simulink model "Debug_STEVAL_BMS _114"  (R2025b)
settings: Solver=FixedStepAuto  StartTime=0.0  StopTime=inf  MaxStep=.01  RelTol=1e-3  EnableMultiTasking=on
PreLoadFcn:
  | %setup_sil;
  | setup_pil;
InitFcn:
  | battery_init;
  | Full_Charge_Volt=4.2; % unit volts
  | Cutoff_Volt=3; % unit volts
  | Delta=.02;
  | ContactorTime=20;
  | ContactorTimeOut=100;
  | High_TempLim=333;
  | Low_TempLim=263;
  | Sensor_Fault_Treshold=.02;
  | CurrentTimeout=1;
  | Allowed_Delta=.04;
  | Bal_On_Time=30;
  | Bal_Off_Time=5;
  | BalNotAct_Time=10;
libraries: simulink x7, stm32blockslib x1, stm32f4xxblockslib x1
settings Model: DataDictionary=Needed_Buses.sldd  STM32="{\"DigitalPortWrite\":[{\"ID\":\"MCU_CODE:12\"},{\"ID\":\"MCU_CODE_Copy:132\"},{\"ID\":\"BMS_PIL_Wrapper:132\"},{\"ID\":\"BMS_MCU_CODE:1376\"}],\"DigitalPortRead\":[{\"ID\":\"MCU_CODE_Copy:131\"},{\"ID\":\"BMS_PIL_Wrapper:131\"}],\"SPIControllerTransfer\":{\"ID\":\"BMS_MCU_CODE:732\"}}"  SILPILSystemUnderTest=refmodels  CodeVerificationMode=processor-in-the-loop (pil)  Creator=Odonata-KJ  LastModifiedBy=Odonata-KJ
settings SolverCC: AutoInsertRateTranBlk=on
settings DataIOCC: SaveOutput=off  SaveTime=off
settings OptimizationCC: EnhancedBackFolding=on  PassReuseOutputArgsAs=Individual arguments  ZeroExternalMemoryAtStartup=off  ZeroInternalMemoryAtStartup=off  MaxStackSize=512  OptimizeBlockOrder=speed  DifferentSizesBufferReuse=on  OptimizationCustomize=off  EfficientTunableParamExpr=on
settings DebuggingCC: ParameterTunabilityLossMsg=error  SFUnexpectedBacktrackingDiag=warning  SFNoUnconditionalDefaultTransitionDiag=warning  UnderSpecifiedDimensionMsg=warning
settings HardwareCC: ProdBitPerPointer=32.0  ProdBitPerSizeT=32.0  ProdBitPerPtrDiffT=32.0  ProdLargestAtomicInteger=Long  ProdLargestAtomicFloat=Double  ProdWordSize=32.0  ProdLongLongMode=on  ProdHWDeviceType=ARM Compatible->ARM Cortex-M  TargetLargestAtomicInteger=Long  TargetLargestAtomicFloat=Double  TargetIntDivRoundTo=Zero  TargetEndianess=LittleEndian  TargetHWDeviceType=ARM Compatible->ARM Cortex-M
settings SFSimCC: MATLABDynamicMemAlloc=off
settings RTWCC: SystemTargetFile=ert.tlc  HardwareBoard=STM32F4xx Based  TemplateMakefile=ert_default_tmf  GenerateReport=on  Toolchain=GNU Tools for ARM Embedded Processors  BuildConfiguration=Debug  LaunchReport=on  PortableWordSizes=on  Description=Embedded Coder
settings CodeAppCC: ForceParamTrailComments=on  IgnoreCustomStorageClasses=off  OperatorAnnotations=on  SimulinkDataObjDesc=on  SFDataObjDesc=on  InsertBlockDesc=on  EnableCustomComments=on
settings ERTTargetCC: ExtModeTransport=3.0  ExtModeStaticAlloc=on  ExtModeStaticAllocSize=2048.0  ExtModeMexFile=ext_xcp  ExtModeIntrfLevel=Level2 - Open  InlinedParameterPlacement=Hierarchical  TargetLangStandard=C99 (ISO)

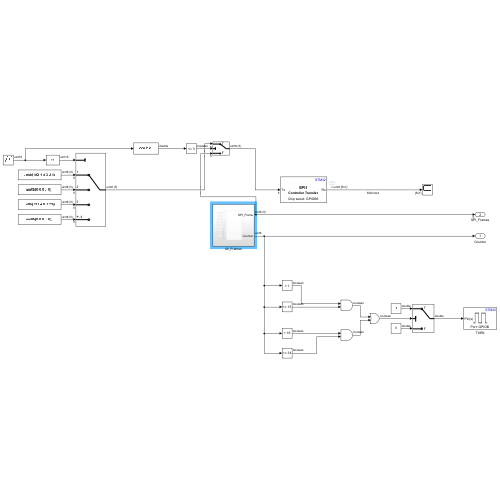
[thumbnail: Simulink's stored preview of the top-level diagram]
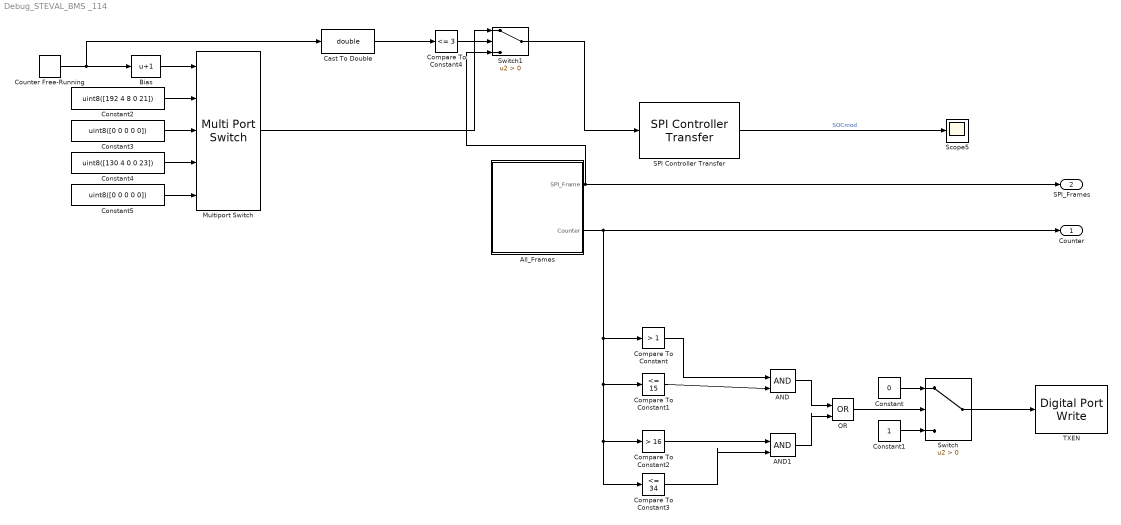
== system Debug_STEVAL_BMS _114 ==
  AND : Logic  IconShape=distinctive  AllPortsSameDT=off  OutDataTypeStr=boolean
  AND1 : Logic  IconShape=distinctive  AllPortsSameDT=off  OutDataTypeStr=boolean
  All_Frames : Subsystem
  Bias : Bias  Bias=1  SaturateOnIntegerOverflow=off
  Cast To Double : DataTypeConversion  OutDataTypeStr=double  SaturateOnIntegerOverflow=off  RndMeth=Floor
  Compare To Constant : simulink/Logic and Bit Operations/Compare To Constant  relop=>  const=1  OutDataTypeStr=boolean
  Compare To Constant1 : simulink/Logic and Bit Operations/Compare To Constant  relop=<=  const=15  OutDataTypeStr=boolean
  Compare To Constant2 : simulink/Logic and Bit Operations/Compare To Constant  relop=>  const=16  OutDataTypeStr=boolean
  Compare To Constant3 : simulink/Logic and Bit Operations/Compare To Constant  relop=<=  const=34  OutDataTypeStr=boolean
  Compare To Constant4 : simulink/Logic and Bit Operations/Compare To Constant  relop=<=  const=3  OutDataTypeStr=boolean
  Constant : Constant  Value=0
  Constant1 : Constant
  Constant2 : Constant  Value=uint8([192 4 8 0 21])
  Constant3 : Constant  Value=uint8([0 0 0 0 0])
  Constant4 : Constant  Value=uint8([130 4 0 0 23])
  Constant5 : Constant  Value=uint8([0 0 0 0 0])
  Counter Free-Running : simulink/Sources/Counter Free-Running  NumBits=16  tsamp=-1
  Multiport Switch : MultiPortSwitch  Inputs=4  SaturateOnIntegerOverflow=off  InputSameDT=off
  OR : Logic  Operator=OR  IconShape=distinctive  AllPortsSameDT=off  OutDataTypeStr=boolean
  SPI Controller Transfer : stm32blockslib/SPI Controller Transfer  SPIModuleSelect=SPI1  ClockPolarity=Low  ClockPhase=1 Edge  SPIModule=uint32(0)  Mode=Master  BusSpeed=uint32(1000000)  FirstBitToTransfer=Most significant bit (MSB)  ClockMode=0  BlockFunction=Transfer  EnableRegisterAddress=off  RegisterAddress=0  OutputDataType=uint8  OutputDataLength=1  OutputStatus=off  BlockingMode=off  Timeout=0.001  DataBits=8  UseCustomSSPin=Explicit GPIO calls  ActiveLowSSPin=Active low  Port_Select=GPIOB  Pin=6
      settings: LibrarySourceBlock=stm32f4xxblockslib/SPI Controller Transfer
  Scope5 : Scope
      settings: DataLoggingVariableName=ScopeData5
  Switch : Switch  Criteria=u2 > Threshold  SaturateOnIntegerOverflow=off  InputSameDT=off
  Switch1 : Switch  Criteria=u2 > Threshold  SaturateOnIntegerOverflow=off  InputSameDT=off
  TXEN : stm32f4xxblockslib/Digital Port Write  PortName=GPIOB  PinNumber=[5]  ReadOperation=off  IOAsArray=on  EnableSimPort=off  hoistedMaskSrc=ECSoC/ECSimCodegen/Digital Port Write
  Counter : Outport
  SPI_Frames : Outport  Port=2
  wires:
  SPI Controller Transfer/1 -> Scope5/1  "SOCmod"
  Constant2/1 -> Multiport Switch/2
  Constant3/1 -> Multiport Switch/3
  Constant4/1 -> Multiport Switch/4
  Constant5/1 -> Multiport Switch/5
  Bias/1 -> Multiport Switch/1
  Counter Free-Running/1 -> Cast To Double/1, Bias/1
  Switch/1 -> TXEN/1
  Constant/1 -> Switch/1
  Compare To Constant2/1 -> AND1/1
  All_Frames/1(SPI_Frame) -> Switch1/3, SPI_Frames/1
  AND1/1 -> OR/2
  Constant1/1 -> Switch/3
  AND/1 -> OR/1
  Compare To Constant/1 -> AND/1
  Compare To Constant3/1 -> AND1/2
  Compare To Constant1/1 -> AND/2
  All_Frames/2(Counter) -> Compare To Constant2/1, Compare To Constant3/1, Compare To Constant1/1, Compare To Constant/1, Counter/1
  Cast To Double/1 -> Compare To Constant4/1
  Switch1/1 -> SPI Controller Transfer/1
  Multiport Switch/1 -> Switch1/1
  Compare To Constant4/1 -> Switch1/2
  OR/1 -> Switch/2

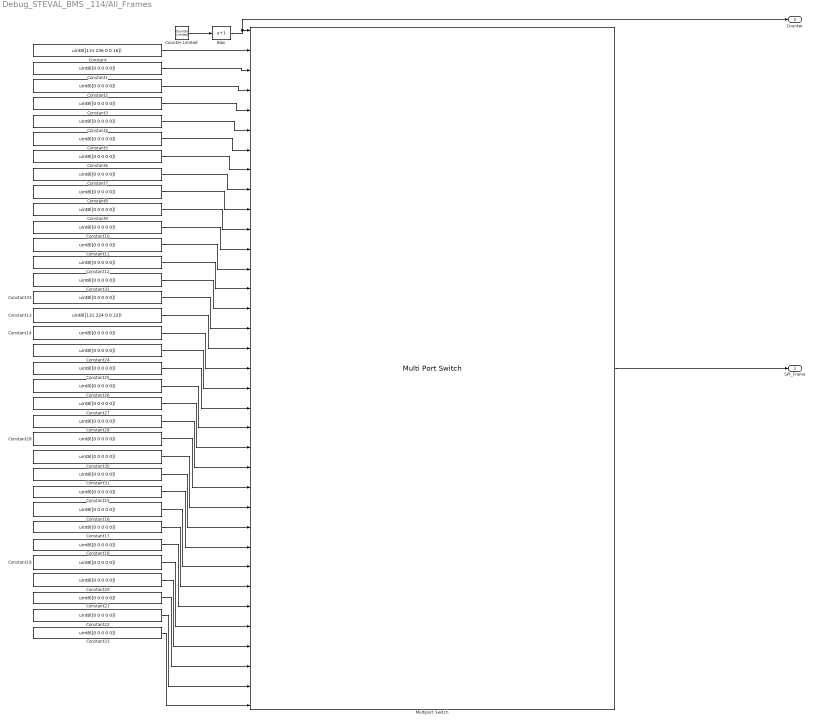
== system Debug_STEVAL_BMS _114/All_Frames ==
  Bias : Bias  Bias=1  SaturateOnIntegerOverflow=off
  Constant : Constant  Value=uint8([131 236 0 0 16])
  Constant{1..12,14..33} (32 alike) : Constant  Value=uint8([0 0 0 0 0])
  Constant13 : Constant  Value=uint8([131 224 0 0 22])
  Counter Limited : simulink/Sources/Counter Limited  uplimit=37  tsamp=-1
  Multiport Switch : MultiPortSwitch  Inputs=34  OutDataTypeStr=uint8  SaturateOnIntegerOverflow=off  InputSameDT=off
  SPI_Frame : Outport
  Counter : Outport  Port=2
  wires:
  Multiport Switch/1 -> SPI_Frame/1
  Counter Limited/1 -> Bias/1
  Bias/1 -> Multiport Switch/1, Counter/1
  Constant/1 -> Multiport Switch/2
  Constant1/1 -> Multiport Switch/3
  Constant2/1 -> Multiport Switch/4
  Constant3/1 -> Multiport Switch/5
  Constant4/1 -> Multiport Switch/6
  Constant5/1 -> Multiport Switch/7
  Constant6/1 -> Multiport Switch/8
  Constant7/1 -> Multiport Switch/9
  Constant8/1 -> Multiport Switch/10
  Constant9/1 -> Multiport Switch/11
  Constant10/1 -> Multiport Switch/12
  Constant11/1 -> Multiport Switch/13
  Constant12/1 -> Multiport Switch/14
  Constant33/1 -> Multiport Switch/16
  Constant32/1 -> Multiport Switch/15
  Constant13/1 -> Multiport Switch/17
  Constant14/1 -> Multiport Switch/18
  Constant24/1 -> Multiport Switch/19
  Constant25/1 -> Multiport Switch/20
  Constant26/1 -> Multiport Switch/21
  Constant27/1 -> Multiport Switch/22
  Constant28/1 -> Multiport Switch/23
  Constant29/1 -> Multiport Switch/24
  Constant31/1 -> Multiport Switch/26
  Constant30/1 -> Multiport Switch/25
  Constant15/1 -> Multiport Switch/27
  Constant16/1 -> Multiport Switch/28
  Constant17/1 -> Multiport Switch/29
  Constant18/1 -> Multiport Switch/30
  Constant19/1 -> Multiport Switch/31
  Constant20/1 -> Multiport Switch/32
  Constant21/1 -> Multiport Switch/33
  Constant22/1 -> Multiport Switch/34
  Constant23/1 -> Multiport Switch/35
